simulink model "reactionWheelSim"  (R2025a)
settings: Solver=FixedStepAuto  StartTime=0.0  StopTime=120  FixedStep=.1  RelTol=1e-3
undefined symbols (not defined in the file or in its folder): IAU
libraries: aerolibtransform2 x2, aerolibutil x2
settings Model: Creator=cdwy3  LastModifiedBy=cdwy3

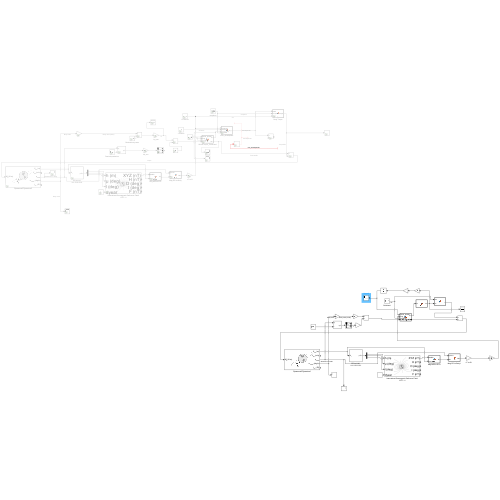
[thumbnail: Simulink's stored preview of the top-level diagram]
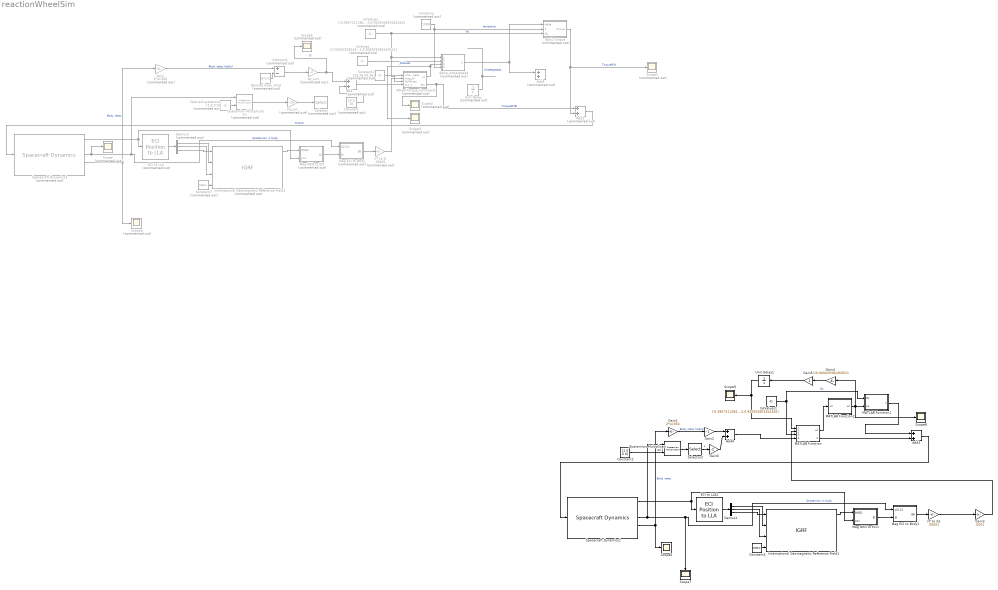
== system reactionWheelSim ==
  Add : Sum  Commented=on
  Add1 : Sum  Commented=on
  Add2 : Sum  Commented=on
  Add3 : Sum
  Add4 : Sum
  Body Torque : MATLAB Function  Commented=on  TreatAsAtomicUnit=on
  Constant : Constant  Commented=on  Value=[0 0 0]
  Constant1 : Constant  Commented=on  Value=[26,26,26,26]
  Constant2 : Constant  Value=[1 0 0 0]
  Constant4 : Constant  Value=2025.2
  Constant7 : Constant  Commented=on  Value=2025.2
  Demux1 : Demux  Outputs=3
  Demux2 : Demux  Commented=on  Outputs=3
  Desired body rates : Constant  Commented=on  Value=[0,0,0]
  Desired quaternion : Constant  Commented=on  Value=[1,0,0,0]
  ECI to LLA : aerolibtransform2/ECI Position to LLA  Commented=on  red=IAU-2000/2006  year=2013  month=January  day=1  hour=0  min=0  sec=0  deltaT=None  errorflag=Error  extraparamflag=off  eunits=Metric (MKS)  earthmodel=WGS84  flat=1/298.257223563  eqradius=6378137
      settings: AttributesFormatString=%<red>
  ECI to LLA1 : aerolibtransform2/ECI Position to LLA  red=IAU-2000/2006  year=2013  month=January  day=1  hour=0  min=0  sec=0  deltaT=None  errorflag=Error  extraparamflag=off  eunits=Metric (MKS)  earthmodel=WGS84  flat=1/298.257223563  eqradius=6378137
      settings: AttributesFormatString=%<red>
  Gain : Gain  Commented=on  Gain=2*pi/360
  Gain1 : Gain  Gain=2*pi/360
  Gain2 : Gain  Gain=-1
  Gain3 : Gain  Gain=.0001
  Gain4 : Gain  Gain=1/0.000029382450521
  Gain5 : Gain  Gain=.1
  Gain6 : Gain  Gain=-2
  GsValues : Constant  Commented=on  Value=[-0.390731128489274,-0.390731128489274,0.390731128489274,0.390731128489274;0.0,0.920504853452440,0.920504853452440,0.0;0.920504853452440,0.0,0.0,0.920504853452440]
  GsValues1 : Constant  Value=[-0.390731128489274,-0.390731128489274,0.390731128489274,0.390731128489274;0.0,0.920504853452440,0.920504853452440,0.0;0.920504853452440,0.0,0.0,0.920504853452440]
  International Geomagnetic Reference Field1 : IGRF  month=January  day=1  sv_out=off
      settings: AttributesFormatString=%<generation>
  International Geomagnetic Reference Field3 : IGRF  Commented=on  month=January  day=1  sv_out=off
      settings: AttributesFormatString=%<generation>
  JsValues : Constant  Commented=on  Value=[0.000029382450521,0.000029382450521,0.000029382450521,0.000029382450521]
  MATLAB Function : MATLAB Function  TreatAsAtomicUnit=on
  MATLAB Function1 : MATLAB Function  TreatAsAtomicUnit=on
  MATLAB Function2 : MATLAB Function  TreatAsAtomicUnit=on
  Mag ECI to Body : MATLAB Function  Commented=on  TreatAsAtomicUnit=on
  Mag ECI to Body1 : MATLAB Function  TreatAsAtomicUnit=on
  Mag NED to ECI : MATLAB Function  Commented=on  TreatAsAtomicUnit=on
  Mag NED to ECI1 : MATLAB Function  TreatAsAtomicUnit=on
  Quaternion Multiplication : aerolibutil/Quaternion Multiplication  Commented=on
  Quaternion Multiplication1 : aerolibutil/Quaternion Multiplication
  Scope{,1..5} (6 alike) : Scope  Commented=on
      Scope settings: ActiveDisplayYMinimum=-1  ActiveDisplayYMaximum=1
      Scope1 settings: ActiveDisplayYMinimum=0.00092159753269089109  ActiveDisplayYMaximum=0.00162242274710922
      Scope2 settings: ActiveDisplayYMinimum=-1  ActiveDisplayYMaximum=1  DataLoggingVariableName=ScopeData2
      Scope3 settings: ActiveDisplayYMinimum=-1  ActiveDisplayYMaximum=1  DataLoggingVariableName=ScopeData3
      Scope4 settings: ActiveDisplayYMinimum=-4.2511925001015065  ActiveDisplayYMaximum=9.4040486463892474  YLabel=Body Rates (deg/s)  DataLoggingVariableName=ScopeData4
      Scope5 settings: ActiveDisplayYMinimum=-0.10478750798382198  ActiveDisplayYMaximum=-0.104671821526179  DataLoggingVariableName=ScopeData5
  Scope{6..9} (4 alike) : Scope
      Scope6 settings: ActiveDisplayYMinimum=-3.3418327171436069  ActiveDisplayYMaximum=4.0650082058708179  DataLoggingVariableName=ScopeData6
      Scope7 settings: ActiveDisplayYMinimum=-0.13544755255044388  ActiveDisplayYMaximum=1.1261608391722715  DataLoggingVariableName=ScopeData9
      Scope8 settings: ActiveDisplayYMinimum=-0.14868626330450829  ActiveDisplayYMaximum=0.800834010540642  DataLoggingVariableName=ScopeData7
      Scope9 settings: ActiveDisplayYMinimum=-14.906936925115286  ActiveDisplayYMaximum=11.855297678315045  DataLoggingVariableName=ScopeData8
  Selector : Selector  Commented=on  InputPortWidth=4  IndexOptions=Index vector (dialog)  Indices=[2 3 4]  OutputSizes=1
  Selector2 : Selector  InputPortWidth=4  IndexOptions=Index vector (dialog)  Indices=[2 3 4]  OutputSizes=1
  Spacecraft Dynamics1 : SpacecraftDynamics  forcesIn=off  startDate=2460438.0  mass=9.0  inertia=[0.0797 -0.00005 0.00125 ;-0.00005 0.1291 -0.00103;0.00125 -0.00103 0.1310]  orbitType=Circular inclined  semiMajorAxis=6821000  eccentricity=0  inclination=55  raan=0  argPeriapsis=0  trueAnomaly=0  attitudeRate=[5 5 5]  useGravGrad=off
  Spacecraft Dynamics3 : SpacecraftDynamics  Commented=on  forcesIn=off  startDate=2460438.0  mass=9.0  inertia=[0.0797 -0.00005 0.00125 ;-0.00005 0.1291 -0.00103;0.00125 -0.00103 0.1310]  orbitType=Circular inclined  semiMajorAxis=6821000  eccentricity=0  inclination=55  raan=0  argPeriapsis=0  trueAnomaly=0  attitudeRate=[0 0 0]  useGravGrad=off
  Subtract1 : Sum  Commented=on  Inputs=+-
  Unit Delay : UnitDelay  Commented=on  InitialCondition=[0;0;0;0]  SampleTime=-1  HasFrameUpgradeWarning=on
  Unit Delay1 : UnitDelay  InitialCondition=[0;0;0;0]  SampleTime=-1  HasFrameUpgradeWarning=on
  WheelTorque_Command : MATLAB Function  Commented=on  TreatAsAtomicUnit=on
  delta_wheelspeed : MATLAB Function  Commented=on  TreatAsAtomicUnit=on
  kd_sun : Gain  Commented=on  Gain=-.10
  kp_sun : Gain  Commented=on  Gain=-2
  nT to G : Gain  Commented=on  Gain=.00001
  nT to G1 : Gain  Gain=.00001
  ramptime : Constant  Commented=on  Value=1000
  wires:
  Constant7/1 -> International Geomagnetic Reference Field3/4
  Spacecraft Dynamics3/1 -> ECI to LLA/1, Mag NED to ECI/2(pos)
  International Geomagnetic Reference Field3/1 -> Mag NED to ECI/1(BNED)
  Mag NED to ECI/1(BI) -> Mag ECI to Body/2(BI)
  Spacecraft Dynamics3/3 -> Scope/1, Quaternion Multiplication/1, Mag ECI to Body/1(q0123)  "Quaternion in body"
  Mag ECI to Body/1(BB) -> nT to G/1
  nT to G/1 -> WheelTorque_Command/2(mag_bf)
  Spacecraft Dynamics3/4 -> Scope4/1, Gain/1  "Body rates"
  ECI to LLA/1 -> Demux2/1
  Demux2/1 -> International Geomagnetic Reference Field3/2
  Demux2/2 -> International Geomagnetic Reference Field3/3
  Demux2/3 -> International Geomagnetic Reference Field3/1
  Desired body rates/1 -> Subtract1/2
  Gain/1 -> Subtract1/1  "Body rates (rad/s)"
  Subtract1/1 -> kp_sun/1
  kp_sun/1 -> Scope5/1, Add/1  "D"
  Add/1 -> WheelTorque_Command/4(out_u)
  GsValues/1 -> WheelTorque_Command/3(GsValues), delta_wheelspeed/1(GsValues), Body Torque/3(Gs)  "Gs"
  ramptime/1 -> delta_wheelspeed/4(rampMS), Body Torque/2(rampMS)  "ramptime"
  JsValues/1 -> delta_wheelspeed/2(JsValues)  "JsValues"
  Unit Delay/1 -> ?  "wheelspeeds"
  WheelTorque_Command/2(tau) -> Scope2/1, Add2/1  "TorqueMTB"
  Add2/1 -> Spacecraft Dynamics3/1  "torque"
  ? -> Unit Delay/1  "new_wheelspeeds"
  Body Torque/1(torque) -> Scope1/1, Add2/2  "TorqueRW"
  kd_sun/1 -> Selector/1
  delta_wheelspeed/1(del_ws_r) -> Add1/1, Body Torque/1(delta)
  Desired quaternion/1 -> Quaternion Multiplication/2
  Quaternion Multiplication/1 -> kd_sun/1
  Constant1/1 -> WheelTorque_Command/1(wheel_speeds)
  Constant/1 -> Add/2
  WheelTorque_Command/1(us) -> Scope3/1, delta_wheelspeed/3(torque_req)
  Demux1/1 -> International Geomagnetic Reference Field1/2
  Constant4/1 -> International Geomagnetic Reference Field1/4
  Spacecraft Dynamics1/1 -> ECI to LLA1/1, Mag NED to ECI1/2(pos)
  Spacecraft Dynamics1/4 -> Gain1/1, Scope6/1  "Body rates"
  Demux1/3 -> International Geomagnetic Reference Field1/1
  Spacecraft Dynamics1/3 -> Quaternion Multiplication1/1, Scope7/1, Mag ECI to Body1/1(q0123)  "Quaternion in body"
  International Geomagnetic Reference Field1/1 -> Mag NED to ECI1/1(BNED)
  Demux1/2 -> International Geomagnetic Reference Field1/3
  ECI to LLA1/1 -> Demux1/1
  Mag NED to ECI1/1(BI) -> Mag ECI to Body1/2(BI)
  Mag ECI to Body1/1(BB) -> nT to G1/1
  Gain1/1 -> Gain2/1  "Body rates (rad/s)"
  nT to G1/1 -> Gain3/1
  GsValues1/1 -> MATLAB Function/3(GsValues), MATLAB Function1/1(Gs)  "Gs"
  MATLAB Function1/1(t) -> Add3/1
  MATLAB Function/2(tauMTB) -> Add3/2
  Gain3/1 -> MATLAB Function/2(mag_bf)
  Add3/1 -> Spacecraft Dynamics1/1
  MATLAB Function/1(us) -> MATLAB Function2/1("us ")
  MATLAB Function2/1(us) -> Gain4/1, Scope8/1, MATLAB Function1/2(us)
  Gain4/1 -> Gain5/1
  Gain5/1 -> Unit Delay1/1
  Unit Delay1/1 -> MATLAB Function/1(wheel_speeds), Scope9/1
  Gain2/1 -> Add4/1
  Constant2/1 -> Quaternion Multiplication1/2
  Quaternion Multiplication1/1 -> Selector2/1
  Selector2/1 -> Gain6/1  "P"
  Gain6/1 -> Add4/2
  Add4/1 -> MATLAB Function/4(L_R_input)

== matlab function reactionWheelSim/WheelTorque_Command ==
  data: wheel_speeds input; us output; mag_bf input; GsValues input; out_u input; tau output
function [us,tau] = wt(wheel_speeds, mag_bf, GsValues, out_u)

    % RW spin axis inertia
    Iws = 0.000029382450521;
    % Despin gain scaler (make this small so it doesn't dominate)
    c   = 0.00005;     
    
    % Build Gs matrix
    G_s = [ GsValues(1:4) ; 
            GsValues(5:8) ; 
            GsValues(9:12) ];
    
    % Wheel speed bias (rad/s)
    OmegaD = 250*2*pi/60 * ones(4,1); 
    
    % Identity mapping for torque rods
    Gt = eye(3);

    % Convert magnetic field from Gauss → Tesla
    B_field = (mag_bf(:)) * 1e-4;
    
    % Requested control torque from higher-level controller
    L_R = out_u(1:3);  
    
    % Current wheel speeds
    Omega = wheel_speeds(:);
    
    % Magnetic Field skew-symmetric matrix
    B_tilde = [   0        -B_field(3)   B_field(2);
                  B_field(3)    0       -B_field(1);
                 -B_field(2)  B_field(1)    0      ];
    
    %---------------------------------------------------------
    % Pseudo-inverse of Gs
    %---------------------------------------------------------
    Gs_pinv = pinv(G_s);
    
    %---------------------------------------------------------
    % Required RW torque from controller
    % usReq = pinv(Gs) * (-L_R)
    %---------------------------------------------------------
    usReq = Gs_pinv * (-L_R);
    
    %---------------------------------------------------------
    % Small despin / bias correction
    % usStar = -alpha * c * Iws * (Omega - OmegaD)
    %---------------------------------------------------------
    temp_diff = Omega - OmegaD;
    usStar    = -1*c * Iws * temp_diff;
    
    %---------------------------------------------------------
    % Required magnetic dipole for despin
    % muStar = -pinv(Btilde*Gt) * Gs * usStar
    %---------------------------------------------------------
    Btilde_Gt = B_tilde * Gt;
    
    if norm(B_field) > 1e-7   % avoid ill-conditioned inverse in eclipse
        BtildeGt_pinv = pinv(Btilde_Gt);
        muStar = -BtildeGt_pinv * (G_s * usStar);
    else
        muStar = zeros(3,1);
    end

    for i = 1:3
        if(muStar(i)>.100)
            muStar(i) = .100;
        end    
        if(muStar(i)<-.100)
            muStar(i) = -.100;
        end
    end
    
    %---------------------------------------------------------
    % Resulting magnetic torque
    % tauMTB = Btilde * Gt * muStar
    %---------------------------------------------------------
    tau = -Btilde_Gt * muStar;
    
    %---------------------------------------------------------
    % Component of torque not produced by MTB
    % deltaU = pinv(Gs) * (tauMTB - Gs*usStar)
    %---------------------------------------------------------
    temp3  =  (tau-G_s*usStar);%-1* (G_s * usStar)-tauMTB;
    deltaU = Gs_pinv * temp3;
    
    %---------------------------------------------------------
    % Actual applied RW torque
    % us = usReq + usStar - deltaU
    % (note: minus deltaU, per your original comment)
    %---------------------------------------------------------
    us = usReq + usStar + deltaU;
    

end

== matlab function reactionWheelSim/MATLAB Function ==
  data: wheel_speeds input; mag_bf input; GsValues input; L_R_input input; us output; tauMTB output
function [us, tauMTB]  = WheelTorque_Command(wheel_speeds, mag_bf, GsValues, L_R_input)
% MATLAB Function block version of WheelTorque_Command
%
% Inputs:
%   wheel_speeds [4x1]   : Reaction wheel speeds [rad/s]
%   mag_bf       [3x1]   : Magnetic field vector in body frame [T]
%   GsValues     [3x4]   : Wheel geometry / spin axis matrix
%   L_R_input    [3x1]   : Desired control torque from PD controller [Nm]
%
% Output:
%   out_u [7x1] : [us(4x1); tauMTB(3x1)]

    % Constants
    Iws = 0.000029382450521;   % Wheel spin axis inertia [kg·m^2]
    c   = 5;                % Reaction wheel torque to magtorquer scaler
    OmegaD = rpm_to_rads(250) * ones(4,1);  % Desired wheel bias [rad/s]

    % Wheel speed vector
    Omega = wheel_speeds(:);

    % L_R from PD controller
    L_R = L_R_input(:);

    % Torque rod transformation (identity)
    Gt = eye(3);

    % Compute pseudo-inverse of Gs
    Gs = GsValues;
    Gs_pinv = pinv(Gs);

    % RW torque required to track commanded torque
    usReq = Gs_pinv * (-L_R);

    % Despin torque
    usStar = -c * Iws * (Omega - OmegaD);

    % Skew-symmetric matrix of magnetic field
    B_tilde = [   0      -mag_bf(3)  mag_bf(2);
               mag_bf(3)     0      -mag_bf(1);
              -mag_bf(2)  mag_bf(1)     0     ];

     
    Btilde_Gt = B_tilde * Gt;
    muStar = -pinv(Btilde_Gt) * Gs * usStar;
    for i = 1:3
        if(muStar(i)>.1)
            muStar(i) = .1;
        end
        if(muStar(i)<-.1)
            muStar(i) = -.1;
        end
    end

    % Magnetic torque
    tauMTB = -(Btilde_Gt) * muStar;

    % deltaU = pinv(Gs) * (tauMTB - Gs*usStar)
    deltaU = Gs_pinv * (tauMTB - Gs * usStar);

    % Actual applied RW torque
    us = usReq + usStar + deltaU;

end

% Helper: RPM to rad/s
function rad_s = rpm_to_rads(rpm)
    rad_s = rpm * (2*pi/60);
end

== matlab function reactionWheelSim/Mag NED to ECI ==
  data: BNED input; BI output; pos input
function BI = NED2I(BNED,pos)

rvec = [pos(1); pos(2); pos(3)];
rho = norm(rvec);

phi=0;
theta = acos(pos(3) / rho);
psi = atan2(pos(2), pos(1));

ct = cos(theta);
st = sin(theta);
sp = sin(phi);
cp = cos(phi);
ss = sin(psi);
cs = cos(psi);

BI = [ct*cs,sp*st*cs-cp*ss,cp*st*cs+sp*ss;
    ct*ss,sp*st*ss+cp*cs,cp*st*ss-sp*cs;
    -st,sp*ct,cp*ct] * BNED;

== matlab function reactionWheelSim/delta_wheelspeed ==
  data: GsValues input; JsValues input; torque_req input; rampMS input; del_ws_r output
function del_ws_r   = d(GsValues, JsValues, torque_req, rampMS)

    % ---- constants ----
    US_MAX = 0.0032; % [Nm] max torque per wheel
    ramptime = rampMS / 1000; % seconds

    % ---- Step 4: Torque saturation ----
    u_s = torque_req(:);
    u_s = max(min(u_s, US_MAX), -US_MAX);

    % ---- Step 5: Torque -> angular acceleration ----
    rw_ang_acc = u_s(:) ./ JsValues(:);

    % ---- Step 6: Integrate over ramp time ----
    del_ws_r = rw_ang_acc * ramptime; % rad/s

    % ---- Step 7: Convert rad/s -> deci-RPM ----
    del_ws = del_ws_r*60/2/pi*10;
    %disp(delta_wheelspeed);

end

== matlab function reactionWheelSim/Body Torque ==
  data: torque output; delta input; rampMS input; Gs input
function torque = torq(delta,rampMS,Gs)

JsValues = [0.000029382450521,0.000029382450521,0.000029382450521,...
			0.000029382450521];
omegadot=delta/(rampMS/1000);
%omegadot_rad_s2 = omegadot * conv_factor;  % 4x1

    % 3) Wheel torques (Nm): u_s = J * omegadot (elementwise)
    torque = -Gs*(JsValues(:) .* omegadot(:));


end

== matlab function reactionWheelSim/Mag ECI to Body1 ==
  data: q0123 input; BB output; BI input
function BB = I2B(q0123,BI)
%compute R such that v(inertial) = TIB v(body)

q0 = q0123(1);
q1 = q0123(2);
q2 = q0123(3);
q3 = q0123(4);

BB = [(q0^2+q1^2-q2^2-q3^2) 2*(q1*q2-q0*q3)  2*(q0*q2+q1*q3);
      2*(q1*q2+q0*q3) (q0^2-q1^2+q2^2-q3^2) 2*(q2*q3-q0*q1);
      2*(q1*q3-q0*q2) 2*(q0*q1+q2*q3) (q0^2-q1^2-q2^2+q3^2)]' * BI;
% Matrix originally adopted from Boom 2010 - Mark Costello
% Copyright - Carlos Montalvo 2015
% You may freely distribute this file but please keep my name in here
% as the original owner

== matlab function reactionWheelSim/Mag ECI to Body ==
  data: q0123 input; BB output; BI input
function BB = I2B(q0123,BI)
%compute R such that v(inertial) = TIB v(body)

q0 = q0123(1);
q1 = q0123(2);
q2 = q0123(3);
q3 = q0123(4);

BB = [(q0^2+q1^2-q2^2-q3^2) 2*(q1*q2-q0*q3)  2*(q0*q2+q1*q3);
      2*(q1*q2+q0*q3) (q0^2-q1^2+q2^2-q3^2) 2*(q2*q3-q0*q1);
      2*(q1*q3-q0*q2) 2*(q0*q1+q2*q3) (q0^2-q1^2-q2^2+q3^2)]' * BI;
% Matrix originally adopted from Boom 2010 - Mark Costello
% Copyright - Carlos Montalvo 2015
% You may freely distribute this file but please keep my name in here
% as the original owner

== matlab function reactionWheelSim/Mag NED to ECI1 ==
  data: BNED input; BI output; pos input
function BI = NED2I(BNED,pos)

rvec = [pos(1); pos(2); pos(3)];
rho = norm(rvec);

phi=0;
theta = acos(pos(3) / rho);
psi = atan2(pos(2), pos(1));

ct = cos(theta);
st = sin(theta);
sp = sin(phi);
cp = cos(phi);
ss = sin(psi);
cs = cos(psi);

BI = [ct*cs,sp*st*cs-cp*ss,cp*st*cs+sp*ss;
    ct*ss,sp*st*ss+cp*cs,cp*st*ss-sp*cs;
    -st,sp*ct,cp*ct] * BNED;

== matlab function reactionWheelSim/MATLAB Function1 ==
  data: Gs input; t output; us input
function t = fcn(Gs,us)

t = -Gs*us;

== matlab function reactionWheelSim/MATLAB Function2 ==
  data: us input; us output
function us = fcn(us)

for i = 1:4
    if(us(i)>.0032)
        us(i) = .0032;
    end
    if(us(i)<.0032)
        us(i)=-.0032;
    end
end
